simulink model "OwenWork"  (R2023a)
settings: Solver=ode45  StartTime=0.0  StopTime=60  RelTol=1e-8  AbsTol=1e-8
undefined symbols (not defined in the file): epsc, etac, I, juliandate, kd, kp, X0
settings Model: Creator=Josh2  LastModifiedBy=Josh2
settings ModelReferenceCC: EnableRefExpFcnMdlSchedulingChecks=on

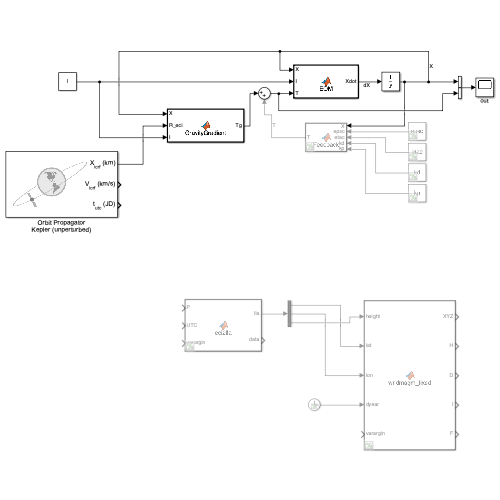
[thumbnail: Simulink's stored preview of the top-level diagram]
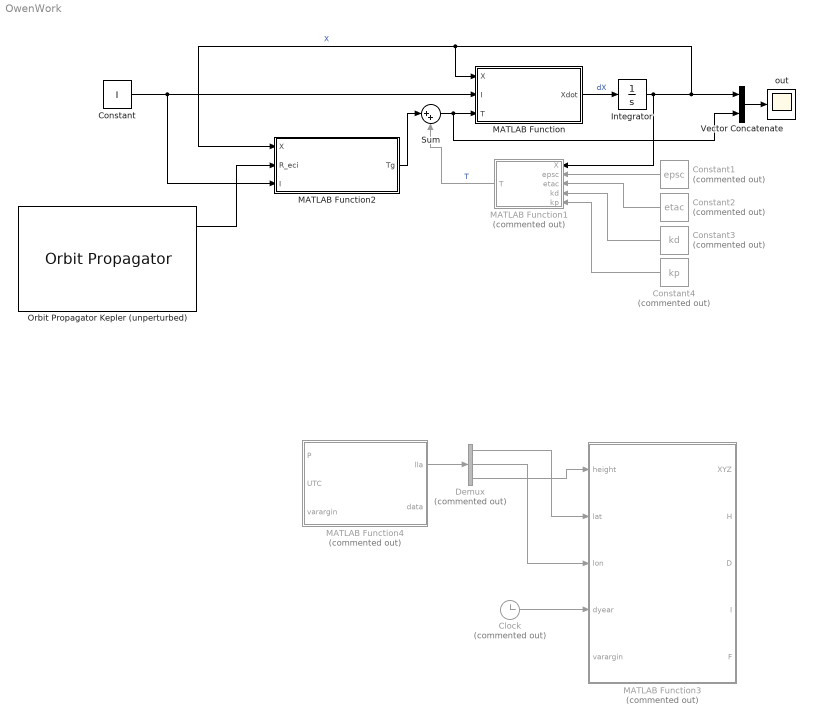
== system OwenWork ==
  Clock : Clock  Commented=on
  Constant : Constant  Value=I
  Constant1 : Constant  Commented=on  Value=epsc
  Constant2 : Constant  Commented=on  Value=etac
  Constant3 : Constant  Commented=on  Value=kd
  Constant4 : Constant  Commented=on  Value=kp
  Demux : Demux  Commented=on  Outputs=3
  Integrator : Integrator  InitialCondition=X0
  MATLAB Function : MATLAB Function  TreatAsAtomicUnit=on
  MATLAB Function1 : MATLAB Function  Commented=on  TreatAsAtomicUnit=on
  MATLAB Function2 : MATLAB Function  TreatAsAtomicUnit=on
  MATLAB Function3 : MATLAB Function  Commented=on  TreatAsAtomicUnit=on
  MATLAB Function4 : MATLAB Function  Commented=on  TreatAsAtomicUnit=on
  Orbit Propagator Kepler (unperturbed) : OrbitPropagator  startDate=juliandate(2023, 6, 21, 8, 0, 0)  semiMajorAxis=7136.6  inertialPosition=[3649700.0 3308200.0 -4676600.0]  inertialVelocity=[-2750.8 6666.4 2573.4]  fixedPosition=[-4142689.0 -2676864.7 -4669861.6]  fixedVelocity=[1452.7 -6720.7 2568.1]  customR=3396200  customMu=4.305e13  customJ2=1.0826269e-03  customOmega=4.06125949e-3  units=Metric (km/s)
  Sum : Sum  Inputs=|++
  Vector Concatenate : Concatenate
  out : Scope
  wires:
  MATLAB Function/1(Xdot) -> Integrator/1  "dX"
  Integrator/1 -> MATLAB Function/1(X), MATLAB Function2/1(X), Vector Concatenate/1, MATLAB Function1/1(X)  "X"
  Constant/1 -> MATLAB Function/2(I), MATLAB Function2/3(I)
  MATLAB Function1/1(T) -> Sum/2  "T"
  Vector Concatenate/1 -> out/1
  Constant1/1 -> MATLAB Function1/2(epsc)
  Constant2/1 -> MATLAB Function1/3(etac)
  Constant3/1 -> MATLAB Function1/4(kd)
  Constant4/1 -> MATLAB Function1/5(kp)
  MATLAB Function2/1(Tg) -> Sum/1
  Sum/1 -> MATLAB Function/3(T), Vector Concatenate/2
  Orbit Propagator Kepler (unperturbed)/1 -> MATLAB Function2/2(R_eci)
  Demux/3 -> MATLAB Function3/1(height)
  Demux/2 -> MATLAB Function3/3(lon)
  MATLAB Function4/1(lla) -> Demux/1
  Demux/1 -> MATLAB Function3/2(lat)
  Clock/1 -> MATLAB Function3/4(dyear)

== matlab function OwenWork/MATLAB Function1 ==
  data: X input; T output; epsc input; etac input; kd input; kp input
function T = Feedback(X,epsc,etac,kd,kp)

% pass through for feedback function

T = zeros(3,1);
T = FEEDBACK_ODE(X,epsc,etac,kd,kp);
end

== matlab function OwenWork/MATLAB Function ==
  data: Xdot output; X input; I input; T input
function Xdot = EOM(X,I,T)
% pass through function calls shared ODE (because this is the world we live in)
Xdot = zeros(10,1);
Xdot = EOM_ODE(0,X,I,T);
end

== matlab function OwenWork/MATLAB Function2 ==
  data: Tg output; X input; R_eci input; I input
function Tg = GravityGradient(X,R_eci,I)
eps = X(7:9);
eta = X(10);

Tg = gravgrad(eps,eta,R_eci,I); 

end

== matlab function OwenWork/MATLAB Function3 ==
  data: height input; XYZ output; lat input; lon input; dyear input; varargin input; H output; D output; I output; F output
function [XYZ, H, D, I, F] = wrldmagm_fixed(height, lat, lon, dyear, varargin)

[XYZ, H, D, I, F] = wrldmagm_fixed(height, lat, lon, dyear, varargin);

end

== matlab function OwenWork/MATLAB Function4 ==
  data: P input; lla output; UTC input; varargin input; data output
function [lla,data] = eci2lla(P,UTC,varargin)

lla = eci2lla(P,UTC,varargin);

end
